simulink model "targetModel"  (R2016b)
settings: Solver=ode4  StartTime=0.0  StopTime=Inf  FixedStep=0.025  RelTol=1e-3  EnableMultiTasking=on
StartFcn:
  | fprintf('\nModel started\n')
  | % Change to root path of simulink model
  | %cd('C:\Users\Doctor V\Desktop\Water Channel Control2');
StopFcn:
  | fprintf('\nModel stopped, running callback.\n')
  | 
  | % change to the home directory
  | fprintf('\nChanging working directory to home directory.\n')
  | %cd('C:\Users\Doctor V\Desktop\Water Channel Control2');
  | 
  | % Add subdirectories to search path
  | fprintf('\nAdding subdirectories to search path.\n')
  | %addpath(genpath(pwd));
  | 
  | % Run stop script to save data and stuff.
  | fprintf('\nRunning stop script ".\\functions\\runAfterSim".\n')
  | %runAfterSim
model workspace (MAT data in the model file):
  Ts = 0.025
undefined symbols (not defined in the file or in its folder): acA2000, Ace, Basler, Freerun_FIX_YAW, PoCL
libraries: slrtlib x4, xpcbitflowlib x3, xpcvideoutillib x2, xpcnilib x1, xpcrtudplib x1
(part 1 of 3)
settings Model: xpc_rtwmakecfg_data=_jpeg__bitflow_  SimulationMode=external  Creator=gweast  LastModifiedBy=Doctor V
settings SolverCC: EnableConcurrentExecution=on
settings DataIOCC: MaxDataPoints=9999999999999999999999999999  SaveFormat=Array  SignalLoggingSaveFormat=ModelDataLogs  SaveState=on  SignalLogging=off  DSMLogging=off  VisualizeSimOutput=off
settings OptimizationCC: BlockReduction=off  OptimizeBlockIOStorage=off  BufferReuse=off  GlobalBufferReuse=off  ExpressionFolding=off  ExpressionDepthLimit=2147483647  LocalBlockOutputs=off  LifeSpan=inf  SimCompilerOptimization=on
settings DebuggingCC: UnderspecifiedInitializationDetection=Classic  MergeDetectMultiDrivingBlocksExec=none  SolverPrmCheckMsg=warning  FcnCallInpInsideContextMsg=warning  AllowSymbolicDim=off  StateNameClashWarn=warning  SFUnexpectedBacktrackingDiag=warning  SFNoUnconditionalDefaultTransitionDiag=warning  SFExecutionAtInitializationDiag=none
settings HardwareCC: ProdBitPerPointer=32  ProdBitPerSizeT=32  ProdBitPerPtrDiffT=32  ProdLargestAtomicFloat=None  ProdWordSize=32  ProdLongLongMode=on  ProdHWDeviceType=Generic->32-bit x86 compatible  TargetBitPerLong=64  TargetBitPerPointer=64  TargetIntDivRoundTo=Zero  TargetEndianess=LittleEndian  TargetWordSize=64  TargetHWDeviceType=Intel->x86-64
settings ModelReferenceCC: PropagateSignalLabelsOutOfModel=off
settings RTWCC: SystemTargetFile=slrt.tlc  TLCOptions=-axPCModelStackSizeKB=512  TemplateMakefile=slrt_default_tmf  Description=Simulink Real-Time  GenerateReport=on  RTWCompilerOptimization=on
settings ConfigComp: CovMetricSettings=dw  CovHtmlReporting=on  CovSaveCumulativeToWorkspaceVar=on  CovSaveSingleToWorkspaceVar=on  CovExternalEMLEnable=off

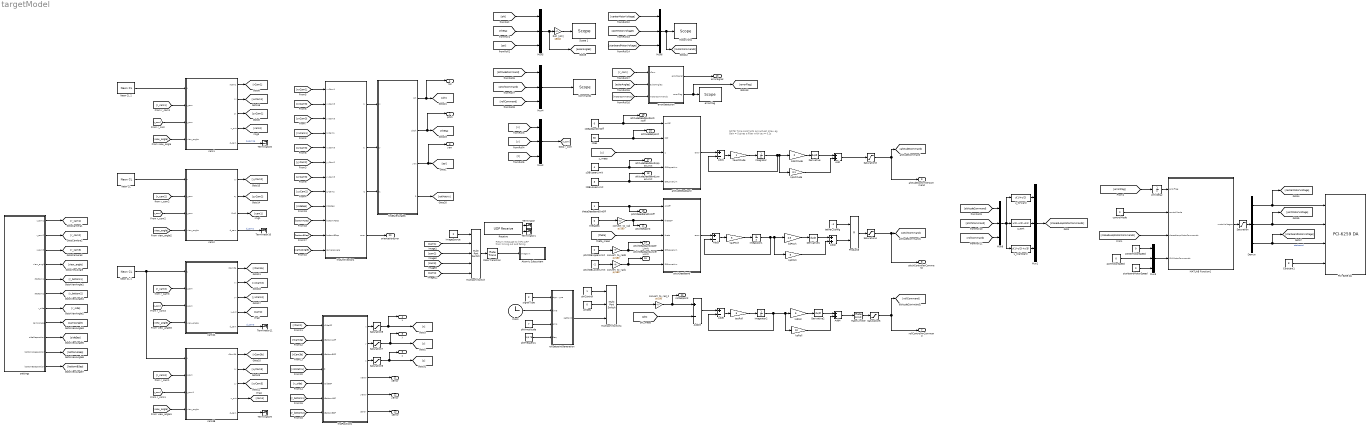
== system targetModel ==
  note: NOTE: Time constants are actuall 1/tau.
      | eg Gain = 5 gives a filter with tau = 0.2s
  note: Return message to keep ARP
      | from timing out and failing
  Add : Sum
  Add{1,3,5,19} (4 alike) : Sum  Inputs=+-
  Add2 : Sum
  Add4 : Sum
  Atomic Subsystem : Subsystem  TreatAsAtomicUnit=on  SystemSampleTime=Ts*3
  Clock : Clock
  Commands : slrtlib/Displays and Logging/Scope   Tag=Power Factor  Priority=1  scopeno=4  scopetype=Target  autostart=on  viewmode=Graphical rolling  formatstr='%15.6f'  grid=on  ylimits=[-1.65,1.65]  nosamples=400  noprepostsamples=0  interleave=1  triggermode=FreeRun  triggersignal=1  trigsignalfromport=off  triggerlevel=0.0  triggerslope=Either  triggerscope=1  triggersample=0  filename=data.dat  mode=Lazy  writesize=512  autorestart=off  dynamicfilemode=off  maxwritefilesize=512*1024^2
  Constant1 : Constant  Value=8
  Demux : Demux  Outputs=3
  Derivative : Derivative
  Derivative1 : Derivative
  Derivative2 : Derivative
  Integrator : Integrator
  Integrator1 : Integrator
  Integrator2 : Integrator
  MATLAB Function1 : MATLAB Function  TreatAsAtomicUnit=on
  "MotorVolts " : slrtlib/Displays and Logging/Scope   Tag=Motor Volts  Priority=2  scopeno=1  scopetype=Target  autostart=on  viewmode=Graphical rolling  formatstr='%15.6f'  grid=on  ylimits=[0,3.3]  nosamples=400  noprepostsamples=0  interleave=1  triggermode=FreeRun  triggersignal=1  trigsignalfromport=off  triggerlevel=0.0  triggerslope=Either  triggerscope=1  triggersample=0  filename=data.dat  mode=Lazy  writesize=512  autorestart=off  dynamicfilemode=off  maxwritefilesize=512*1024^2
  Multiport Switch : MultiPortSwitch  DataPortOrder=Zero-based contiguous  Inputs=4
  Multiport Switch4 : MultiPortSwitch  Inputs=2
  Mux{1..6,8} (7 alike) : Mux  Inputs=3
  "Neon CL " : xpcbitflowlib/Neon CL   camerapath=Basler-Ace-acA2000-340km-PoCL-3Tap-Freerun_FIX - ROLL.r64  r64=CAMERA  sampletime=-1  slot=[7,12]  make=Basler  model=acA2000-340km  mode=3 tap, 8-bits, 2040x1088 PoCL Free running  owner=BitFlow  revision=1  modelcomp=0  revcomp=0  aqtimeout=61440  format=1  flashmux=Mux_2TOEP  flashdcc=DCC  pixbitdepth=8  xsize=2040  ysize=1088  xstart=0  ystart=0  dx=2040  dy=1088  expmod="[0  0]"  config="[4294967295         128;4294967295           0;4294967295         512;4294967295           0;4294967295           0;4294967295           0;4294967295      262144;4294967295           0;4294967295           0;4294967295           0;4294967295     4195324;4294967295           0;4294967295           0;4294967295  4294967295;4294967295           0;4294967295           0;4294967295           0;4294967295    16777215;4294967295        1088;4294967295           0;4294967295           0;4294967295    16777215;4294967295           0;4294967295           0;4294967295           0;4294967295           0;4294967295           0;4294967295           0]"  ctab="[6      0     16      1  36880      2     16     96     18     97     16  32768      0]"  qtabmodel="[1   2040  65536]"  trigmode=0  baud=1  bytewidth=4  parity=1  stopbits=1  command="\"\""  response=0  comments=|
      | Three tap camera, 
      | Acquistion acquires 24 bits per clock, 
      | DMA works as 8-bit data
      | Set XSIZE = 3 * ACPL
  Neon CL 1 : xpcbitflowlib/Neon CL   camerapath=Basler-Ace-acA2000-340km-PoCL-3Tap-Freerun_FIX_YAW.r64  r64=CAMERA  sampletime=-1  slot=[4,12]  make=Basler  model=acA2000-340km  mode=3 tap, 8-bits, 2040x1088 PoCL Free running  owner=BitFlow  revision=1  modelcomp=0  revcomp=0  aqtimeout=61440  format=1  flashmux=Mux_2TOEP  flashdcc=DCC  pixbitdepth=8  xsize=2040  ysize=1088  xstart=0  ystart=0  dx=2040  dy=1088  expmod="[0  0]"  config="[4294967295         128;4294967295           0;4294967295         512;4294967295           0;4294967295           0;4294967295           0;4294967295      262144;4294967295           0;4294967295           0;4294967295           0;4294967295     4195324;4294967295           0;4294967295           0;4294967295  4294967295;4294967295           0;4294967295           0;4294967295           0;4294967295     4958209;4294967295        1088;4294967295           0;4294967295           0;4294967295  2164260863;4294967295           0;4294967295           0;4294967295           0;4294967295           0;4294967295     4958208;4294967295           0]"  ctab="[6      0     16      1  36880      2     16     96     18     97     16  32768      0]"  qtabmodel="[1   2040  65536]"  trigmode=0  baud=1  bytewidth=4  parity=1  stopbits=1  command="\"\""  response=0  comments=|
      | Three tap camera, 
      | Acquistion acquires 24 bits per clock, 
      | DMA works as 8-bit data
      | Set XSIZE = 3 * ACPL
  Neon CL 2 : xpcbitflowlib/Neon CL   camerapath=Basler-Ace-acA2000-340km-PoCL-3Tap-Freerun_FIX - PITCH.r64  r64=CAMERA  sampletime=-1  slot=[13,12]  make=Basler  model=acA2000-340km  mode=3 tap, 8-bits, 2040x1088 PoCL Free running  owner=BitFlow  revision=1  modelcomp=0  revcomp=0  aqtimeout=61440  format=1  flashmux=Mux_2TOEP  flashdcc=DCC  pixbitdepth=8  xsize=2040  ysize=1088  xstart=0  ystart=0  dx=2040  dy=1088  expmod="[0  0]"  config="[4294967295         128;4294967295           0;4294967295         512;4294967295           0;4294967295           0;4294967295           0;4294967295      262144;4294967295           0;4294967295           0;4294967295           0;4294967295     4195324;4294967295           0;4294967295           0;4294967295  4294967295;4294967295           0;4294967295           0;4294967295           0;4294967295     7528449;4294967295        1088;4294967295           0;4294967295           0;4294967295           0;4294967295           0;4294967295           0;4294967295           0;4294967295           0;4294967295     7528448;4294967295           0]"  ctab="[6      0     16      1  36880      2     16     96     18     97     16  32768      0]"  qtabmodel="[1   2040  65536]"  trigmode=0  baud=1  bytewidth=4  parity=1  stopbits=1  command="\"\""  response=0  comments=|
      | Three tap camera, 
      | Acquistion acquires 24 bits per clock, 
      | DMA works as 8-bit data
      | Set XSIZE = 3 * ACPL
  PCI-6259 DA : xpcnilib/D//A/M Series/PCI-6259 DA  channel=[1 2 3 4]  range=[5 10 5 10]  reset=[1 1 1 1]  initValue=[0 0 0 0]  sampletime=-1  slot=-1
  Product3 : Product
  Rate Limiter : RateLimiter  RisingSlewLimit=20  FallingSlewLimit=-20  SampleTimeMode=inherited
  Rate Transition : RateTransition
  Receive : xpcrtudplib/UDP Receive  ipAddressVal=Use host-target connection  localPort=25005  rcvWidth=1  rcvFmAny=off  fmAddress=10.10.10.10  sampleTime=Ts
  Roll_[phi] : Gain  Gain=180/pi
  Saturation : Saturate  UpperLimit=3.3  LowerLimit=0
  Saturation3 : Saturate  UpperLimit=1.65  LowerLimit=-1.65
  Saturation4 : Saturate  UpperLimit=1.65  LowerLimit=-1.65
  Saturation5 : Saturate  UpperLimit=1.65  LowerLimit=-1.65
  Saturation6 : Saturate  UpperLimit=90  LowerLimit=10
  Saturation7 : Saturate  UpperLimit=50  LowerLimit=-50
  Saturation8 : Saturate  UpperLimit=100  LowerLimit=-10
  Scope 1 : slrtlib/Displays and Logging/Scope   scopeno=5  scopetype=Target  autostart=on  viewmode=Graphical redraw  formatstr='%15.6f'  grid=on  ylimits=[0,0]  nosamples=250  noprepostsamples=0  interleave=1  triggermode=FreeRun  triggersignal=1  trigsignalfromport=off  triggerlevel=0.0  triggerslope=Either  triggerscope=1  triggersample=0  filename=data.dat  mode=Lazy  writesize=512  autorestart=off  dynamicfilemode=off  maxwritefilesize=512*1024^2
  Terminator{,1,8..11} (6 alike) : Terminator
  Unit Delay : UnitDelay  SampleTime=-1
  altitudeDeadband : MATLAB Function  TreatAsAtomicUnit=on
  cam1 : Subsystem
  cam2 : Subsystem
  cam3A : Subsystem
  cam3B : Subsystem
  centerMotorSpeed : Constant  Value=0
  controlMode : Constant  Value=0
  convert_to_rad : Gain  Gain=pi/180
  convert_to_rad1 : Gain  Gain=pi/180
  convert_to_rad3 : Gain  Gain=pi/180
  convert_to_rad_2 : Gain  Gain=pi/180
  errorDetection : MATLAB Function  TreatAsAtomicUnit=on
  errorFlag : slrtlib/Displays and Logging/Scope   Tag=Motor Volts  Priority=2  scopeno=2  scopetype=Target  autostart=on  viewmode=Graphical rolling  formatstr='%15.6f'  grid=on  ylimits=[0,2]  nosamples=400  noprepostsamples=0  interleave=1  triggermode=FreeRun  triggersignal=1  trigsignalfromport=off  triggerlevel=0.0  triggerslope=Either  triggerscope=1  triggersample=0  filename=data.dat  mode=Lazy  writesize=512  autorestart=off  dynamicfilemode=off  maxwritefilesize=512*1024^2
  findEulerAngles : MATLAB Function  TreatAsAtomicUnit=on
  findPositions : MATLAB Function  TreatAsAtomicUnit=on
  findUnitVectors : MATLAB Function  TreatAsAtomicUnit=on
  imageSource : Constant  Value=2
  kdAltitude : Gain  Gain=0
  kdPitch : Gain  Gain=2.5
  kdRoll : Gain  Gain=5
  kpAltitude : Gain  Gain=0.1
  kpPitch : Gain  Gain=5
  kpRoll : Gain  Gain=10
  phiAmplitude : Constant  Value=7
  phiControl : Constant
  phiDes : Constant  Value=0
  phiFrequency : Constant  Value=1/5.75
  pitchDBLowerLimit : Constant  Value=-2
  pitchDBUpperLimit : Constant  Value=2
  pitchDeadband : MATLAB Function  TreatAsAtomicUnit=on
  portMotorSpeed : Constant  Value=0
  rollSetpointGeneration : MATLAB Function  TreatAsAtomicUnit=on
  settings : Subsystem
  signalType : Constant  Value=2
  starboardMotorSpeed : Constant  Value=0
  tauAltitude : Gain
  tauPitch : Gain  Gain=5
  tauRoll : Gain  Gain=5
  tether_config : Constant  Value=-1
  thetaDeadbandOnOff : Constant
  thetaDes : Constant  Value=0
  u_forward : Fcn  Expr=u(1)+u(2)
  u_port : Fcn  Expr=u(1)-u(2)-u(3)
  u_starboard : Fcn  Expr=u(1)-u(2)+u(3)
  zDBLowerLimit : Constant  Value=3
  zDBUpperLimit : Constant  Value=4
  zDeadbandOnOff : Constant  Value=0
  zDes : Constant  Value=60
  roll : Outport
  pitch : Outport  Port=2
  yaw : Outport  Port=3
  x : Outport  Port=4
  y : Outport  Port=5
  z : Outport  Port=6
  rollControllerCommand : Outport  Port=7
  pitchControllerCommand : Outport  Port=8
  altitudeControllerCommand : Outport  Port=9
  altitudeSetpoint : Outport  Port=10
  pitchSetpoint : Outport  Port=11
  rollSetpoint : Outport  Port=12
  errorSignal : Outport  Port=13
  pitchDeadbandUpperLimit : Outport  Port=14
  pitchDeadbandLowerLimit : Outport  Port=15
  pitchDeadbandOnOff : Outport  Port=16
  altitudeDeadbandUpperLimit : Outport  Port=17
  altitudeDeadbandLowerLimit : Outport  Port=18
  altitudeDeadbandonOnOff : Outport  Port=19
  orientationError : Outport  Port=20
  xError : Outport  Port=21
  yError : Outport  Port=22
  zError : Outport  Port=23
  wires:
  Constant1/1 -> PCI-6259 DA/4
  controlMode/1 -> MATLAB Function1/2(controlMode)
  [phi] -> Add19/2
  [theta] -> pitchDeadband/3(theta)
  cam1/1(rCam1) -> [rCam1]
  cam3A/1(rCam3a) -> [rCam3a]
  Add19/1 -> Add5/1
  Demux/3 -> [starboardMotorVoltage], PCI-6259 DA/3  "starboard"
  Neon CL 1/1 -> cam3B/1(u), cam3A/1("u ")
  cam1/2(xx) -> [xxCam1]
  cam1/3(zx) -> [zxCam1]
  cam3A/2(xx) -> [xxCam3]
  cam3A/3(yx) -> [yxCam3]
  findEulerAngles/2(pitch) -> pitch/1, [theta]
  findEulerAngles/1(roll) -> roll/1, [phi]
  findPositions/2(y) -> Saturation7/1
  findEulerAngles/3(yaw) -> yaw/1, [psi]
  convert_to_rad_2/1 -> Add19/1, rollSetpoint/1
  findPositions/3(z) -> Saturation6/1
  findPositions/1(x) -> Saturation8/1
  Mux8/1 -> u_starboard/1, u_forward/1, u_port/1
  tether_config/1 -> Product3/1
  Product3/1 -> Saturation4/1
  cam3B/2(xy) -> [xyCam3]
  cam3B/3(yy) -> [yyCam3]
  cam2/1(yy) -> [yyCam2]
  cam2/2(zy) -> [zyCam2]
  Neon CL 2/1 -> cam1/1(u)
  cam3B/4("u_out ") -> [cam4]
  cam2/3(Out1) -> [cam1]
  "Neon CL "/1 -> cam2/1("u ")
  cam3A/4(u_out) -> [cam2]
  Mux5/1 -> [eulerAngles], Roll_[phi]/1
  settings/1(r_cam1) -> [r_cam1]
  settings/2("r_cam2 ") -> [r_cam2]
  settings/3(r_cam3) -> [r_cam3]
  [r_cam1] -> cam1/2(r_cam)
  [r_cam3] -> cam3B/2(r_cam)
  [r_cam2] -> cam2/2(r_cam)
  [r_cam3] -> cam3A/2(r_cam)
  [r_com] -> cam3B/3(r_com1)
  [r_com] -> cam2/3("r_com ")
  [r_com] -> cam3A/3("r_com ")
  [r_com] -> cam1/3(r_com)
  cam1/5(d_cam) -> Terminator8/1  "d_cam1a"
  cam2/4(d_cam) -> Terminator10/1  "d_cam2"
  cam3A/5(d_cam) -> Terminator11/1  "d_cam3"
  cam3B/5(d_cam) -> Terminator9/1
  settings/4(view_angle) -> [view_angle]
  [view_angle] -> cam1/4(view_angle)
  [view_angle] -> cam3B/4(view_angle)
  [view_angle] -> cam2/4(view_angle)
  [view_angle] -> cam3A/4(view_angle)
  cam1/4(u_out) -> [cam3]
  phiAmplitude/1 -> rollSetpointGeneration/3(amp)
  phiFrequency/1 -> rollSetpointGeneration/4(freq)
  Multiport Switch4/1 -> convert_to_rad_2/1
  rollSetpointGeneration/1(setPoint) -> Multiport Switch4/3
  phiDes/1 -> Multiport Switch4/2
  phiControl/1 -> Multiport Switch4/1
  thetaDes/1 -> convert_to_rad/1
  Clock/1 -> rollSetpointGeneration/2(time)
  portMotorSpeed/1 -> Mux3/2
  Mux3/1 -> MATLAB Function1/4(GUIMotorCommands)
  signalType/1 -> rollSetpointGeneration/1(signalType)
  Rate Limiter/1 -> Saturation5/1
  Saturation3/1 -> altitudeControllerCommand/1, [altitudeCommand]
  Saturation4/1 -> pitchControllerCommand/1, [pitchCommand]
  Saturation5/1 -> [rollCommand], rollControllerCommand/1
  zDes/1 -> altitudeDeadband/2(zSP), altitudeSetpoint/1
  u_forward/1 -> Mux1/1
  u_port/1 -> Mux1/2
  u_starboard/1 -> Mux1/3
  Mux1/1 -> [closedLoopMotorCommands]
  [closedLoopMotorCommands] -> MATLAB Function1/3(closedLoopMotorCommands)
  centerMotorSpeed/1 -> Mux3/1
  starboardMotorSpeed/1 -> Mux3/3
  MATLAB Function1/1(motorVoltages) -> Saturation/1
  [psi] -> Mux5/3
  [theta] -> Mux5/2
  [phi] -> Mux5/1
  [z] -> Mux2/3
  [y] -> Mux2/2
  [x] -> Mux2/1
  Mux2/1 -> [r_com]
  Saturation6/1 -> z/1, [z]
  Saturation7/1 -> [y], y/1
  Saturation8/1 -> x/1, [x]
  [rollCommand] -> Mux4/3
  [pitchCommand] -> Mux4/2
  [altitudeCommand] -> Mux4/1
  Mux4/1 -> Commands/1
  [rollCommand] -> Mux8/3
  [pitchCommand] -> Mux8/2
  [altitudeCommand] -> Mux8/1
  tauAltitude/1 -> Integrator/1
  kdAltitude/1 -> Derivative/1
  Integrator/1 -> Add1/2, kpAltitude/1, kdAltitude/1
  Derivative/1 -> Add/1
  kpAltitude/1 -> Add/2
  Add1/1 -> tauAltitude/1
  Add/1 -> Saturation3/1
  tauPitch/1 -> Integrator1/1
  kdPitch/1 -> Derivative1/1
  Integrator1/1 -> Add3/2, kpPitch/1, kdPitch/1
  Add2/1 -> Product3/2
  Derivative1/1 -> Add2/1
  kpPitch/1 -> Add2/2
  Add3/1 -> tauPitch/1
  tauRoll/1 -> Integrator2/1
  kdRoll/1 -> Derivative2/1
  Integrator2/1 -> Add5/2, kpRoll/1, kdRoll/1
  Add4/1 -> Rate Limiter/1
  Derivative2/1 -> Add4/1
  kpRoll/1 -> Add4/2
  Add5/1 -> tauRoll/1
  Saturation/1 -> Demux/1
  Demux/2 -> [portMotorVoltage], PCI-6259 DA/2
  Demux/1 -> [centerMotorVoltage], PCI-6259 DA/1
  [starboardMotorVoltage] -> Mux6/3
  [portMotorVoltage] -> Mux6/2
  [centerMotorVoltage] -> Mux6/1
  Mux6/1 -> [motorCommands], "MotorVolts "/1
  settings/5(rBottom1) -> [r_bottom1]
  settings/7(r_side) -> [r_side]
  [eulerAngles] -> errorDetection/2(eulerAngles)
  errorDetection/2(errorFlag) -> [errorFlag], errorFlag/1
  [motorCommands] -> errorDetection/3(motorCommands)
  [r_com] -> errorDetection/1(rCom)
  errorDetection/1(errorSignal) -> errorSignal/1
  pitchDeadband/1(error) -> Add3/1
  [errorFlag] -> Unit Delay/1
  convert_to_rad/1 -> pitchSetpoint/1, pitchDeadband/2(thetaSP)
  pitchDBUpperLimit/1 -> convert_to_rad3/1
  convert_to_rad3/1 -> pitchDeadband/4(DBUpperLim), pitchDeadbandUpperLimit/1
  Unit Delay/1 -> MATLAB Function1/1(errorFlag)
  pitchDBLowerLimit/1 -> convert_to_rad1/1
  convert_to_rad1/1 -> pitchDeadband/5(DBLowerLim), pitchDeadbandLowerLimit/1
  thetaDeadbandOnOff/1 -> pitchDeadbandOnOff/1, pitchDeadband/1(onOff)
  [z] -> altitudeDeadband/3(z)
  zDeadbandOnOff/1 -> altitudeDeadbandonOnOff/1, altitudeDeadband/1(onOff)
  zDBUpperLimit/1 -> altitudeDeadbandUpperLimit/1, altitudeDeadband/4(DBUpperLim)
  zDBLowerLimit/1 -> altitudeDeadbandLowerLimit/1, altitudeDeadband/5(DBLowerLim)
  altitudeDeadband/1(error) -> Add1/1
  [zyCam2] -> findUnitVectors/8(zyCam2)
  [xxCam1] -> findUnitVectors/1(xxCam1)
  [zxCam1] -> findUnitVectors/4(zxCam1)
  [xxCam3] -> findUnitVectors/2(xxCam3)
  [xyCam3] -> findUnitVectors/5(xyCam3)
  [yxCam3] -> findUnitVectors/3(yxCam3)
  [yyCam3] -> findUnitVectors/7(yyCam3)
  [yyCam2] -> findUnitVectors/6(yyCam2)
  [cam2Angle] -> findUnitVectors/12(cameraAngle)
  settings/8(cam2Angle) -> [cam2Angle]
  findUnitVectors/1(rx) -> findEulerAngles/1(rx)
  findUnitVectors/2(ry) -> findEulerAngles/2(ry)
  findUnitVectors/3(rz) -> findEulerAngles/3(rz)
  findUnitVectors/4(error) -> orientationError/1
  settings/6(rBottom2) -> [r_bottom2]
  cam3B/1(rCam3b) -> [rCam3b]
  [rCam1] -> findPositions/1(rSideGF)
  [rCam3a] -> findPositions/2(rBottomAGF)
  [rCam3b] -> findPositions/3(rBottomBGF)
  [r_side] -> findPositions/5(rSideBF)
  [r_bottom1] -> findPositions/6(rBottomABF)
  [r_bottom2] -> findPositions/7(rBottomBBF)
  findPositions/4(xError) -> xError/1
  findPositions/6(zError) -> zError/1
  findPositions/5(yError) -> yError/1
  [bottomBSep] -> findUnitVectors/11(bottomBSep)
  [bottomASep] -> findUnitVectors/10(bottomASep)
  [sideSep] -> findUnitVectors/9(sideSep)
  settings/9(sideSeparation) -> [sideSep]
  settings/10(bottomASeparation) -> [bottomASep]
  settings/11(bottomBSeparation) -> [bottomBSep]
  findEulerAngles/4(R) -> [rotMatrix]
  [rotMatrix] -> findPositions/4(R)
  Roll_[phi]/1 -> Scope 1/1
  Rate Transition/1 -> Atomic Subsystem/1(Image In)
  Receive/1 -> Terminator/1
  Receive/2 -> Terminator1/1
  imageSource/1 -> Multiport Switch/1
  [cam1] -> Multiport Switch/2
  [cam3] -> Multiport Switch/4
  [cam2] -> Multiport Switch/3
  Multiport Switch/1 -> Rate Transition/1
  [cam4] -> Multiport Switch/5

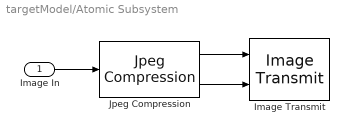
== system targetModel/Atomic Subsystem ==
  Image In : Inport
  Image Transmit : xpcvideoutillib/Image Transmit  ipAddress=255.255.255.255  ipPort=25000  localPort=-1  vblLen=on  maxpacket=40*1024  sampletime=-1
  Jpeg Compression : xpcvideoutillib/Jpeg Compression  quality=35  cspace=Grayscale  isig=One multidimensional signal  maxsize=2040*1088  length=on
  wires:
  Jpeg Compression/1 -> Image Transmit/1
  Jpeg Compression/2 -> Image Transmit/2
  Image In/1 -> Jpeg Compression/1

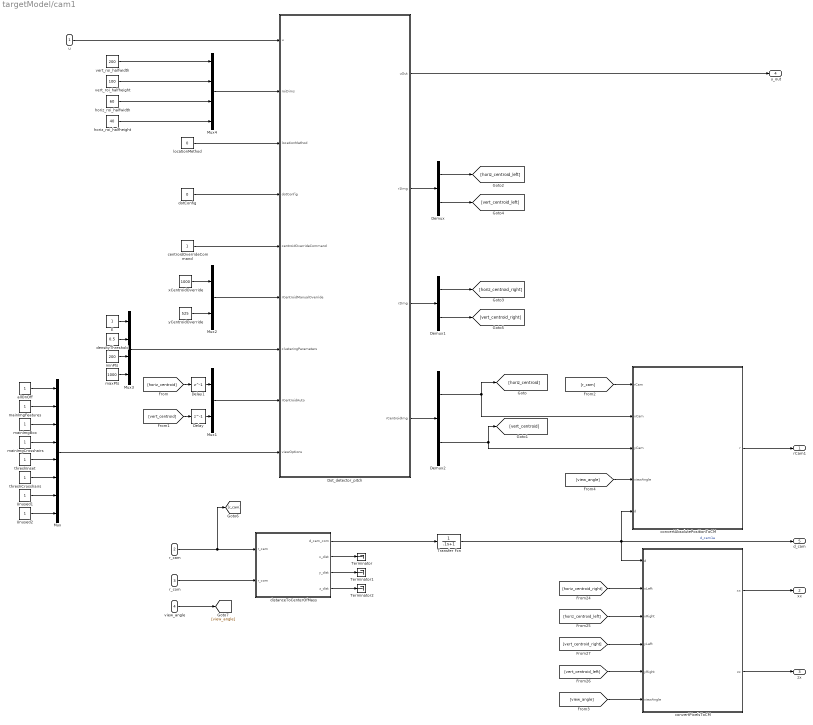
== system targetModel/cam1 ==
  u : Inport
  r_cam : Inport  Port=2
  r_com : Inport  Port=3
  view_angle : Inport  Port=4
  Delay : Delay  DelayLength=1  InitialCondition=800
  Delay1 : Delay  DelayLength=1  InitialCondition=1460
  Demux : Demux  Outputs=2
  Demux1 : Demux  Outputs=2
  Demux2 : Demux  Outputs=2
  Dot_detector_pitch : MATLAB Function  TreatAsAtomicUnit=on
  E : Constant
  Mux : Mux  Inputs=8
  Mux1 : Mux  Inputs=2
  Mux2 : Mux  Inputs=2
  Mux3 : Mux
  Mux4 : Mux
  Terminator : Terminator
  Terminator1 : Terminator
  Terminator2 : Terminator
  Transfer Fcn : TransferFcn  Denominator=[.1 1]
  Unused1 : Constant
  Unused2 : Constant
  allOnOff : Constant
  centroidOverrideCommand : Constant
  convertAbsolutePositionToCM : MATLAB Function  TreatAsAtomicUnit=on
  convertPixelsToCM : MATLAB Function  TreatAsAtomicUnit=on
  densityThreshold : Constant  Value=0.5
  distanceToCenterOfMass : MATLAB Function  TreatAsAtomicUnit=on
  dotConfig : Constant  Value=0
  horiz_roi_halfheight : Constant  Value=40
  horiz_roi_halfwidth : Constant  Value=60
  locationMethod : Constant  Value=0
  mainImgBox : Constant
  mainImgCrosshairs : Constant
  mainImgFeatures : Constant
  maxPts : Constant  Value=1000
  minPts : Constant  Value=200
  threshCrosshairs : Constant
  threshInset : Constant
  vert_roi_halfheight : Constant  Value=100
  vert_roi_halfwidth : Constant  Value=200
  xCentroidOverride : Constant  Value=1000
  yCentroidOverride : Constant  Value=525
  rCam1 : Outport
  xx : Outport  Port=2
  zx : Outport  Port=3
  u_out : Outport  Port=4
  d_cam : Outport  Port=5
  wires:
  [horiz_centroid] -> Delay1/1
  [vert_centroid] -> Delay/1
  allOnOff/1 -> Mux/1
  mainImgFeatures/1 -> Mux/2
  mainImgBox/1 -> Mux/3
  mainImgCrosshairs/1 -> Mux/4
  threshInset/1 -> Mux/5
  threshCrosshairs/1 -> Mux/6
  Unused1/1 -> Mux/7
  Unused2/1 -> Mux/8
  Dot_detector_pitch/1(uOut) -> u_out/1
  Mux1/1 -> Dot_detector_pitch/8(rCentroidAuto)
  Delay1/1 -> Mux1/1
  Delay/1 -> Mux1/2
  xCentroidOverride/1 -> Mux2/1
  yCentroidOverride/1 -> Mux2/2
  densityThreshold/1 -> Mux3/2
  minPts/1 -> Mux3/3
  maxPts/1 -> Mux3/4
  Mux3/1 -> Dot_detector_pitch/7(clusteringParameters)
  E/1 -> Mux3/1
  centroidOverrideCommand/1 -> Dot_detector_pitch/5(centroidOverrideCommand)
  Mux/1 -> Dot_detector_pitch/9(viewOptions)
  u/1 -> Dot_detector_pitch/1(u)
  Mux4/1 -> Dot_detector_pitch/2(roiDims)
  locationMethod/1 -> Dot_detector_pitch/3(locationMethod)
  dotConfig/1 -> Dot_detector_pitch/4(dotConfig)
  Demux/1 -> [horiz_centroid_left]
  Demux/2 -> [vert_centroid_left]
  Dot_detector_pitch/2(r1Img) -> Demux/1
  Dot_detector_pitch/3(r2Img) -> Demux1/1
  Demux1/1 -> [horiz_centroid_right]
  Demux1/2 -> [vert_centroid_right]
  Dot_detector_pitch/4(rCentroidImg) -> Demux2/1
  Demux2/1 -> convertAbsolutePositionToCM/2(xCam), [horiz_centroid]
  Demux2/2 -> convertAbsolutePositionToCM/3(yCam), [vert_centroid]
  Mux2/1 -> Dot_detector_pitch/6(rCentroidManualOverride)
  r_cam/1 -> [r_cam], distanceToCenterOfMass/1(r_cam)
  distanceToCenterOfMass/2(x_dist) -> Terminator/1
  distanceToCenterOfMass/3(y_dist) -> Terminator1/1
  distanceToCenterOfMass/4(z_dist) -> Terminator2/1
  [horiz_centroid_right] -> convertPixelsToCM/2(xLeft)
  [horiz_centroid_left] -> convertPixelsToCM/3(xRight)
  [vert_centroid_right] -> convertPixelsToCM/4(yLeft)
  [vert_centroid_left] -> convertPixelsToCM/5(yRight)
  convertPixelsToCM/1(xx) -> xx/1
  convertPixelsToCM/2(zx) -> zx/1
  r_com/1 -> distanceToCenterOfMass/2(r_com)
  distanceToCenterOfMass/1(d_cam_com) -> Transfer Fcn/1
  Transfer Fcn/1 -> convertAbsolutePositionToCM/5(d), convertPixelsToCM/1(d), d_cam/1  "d_cam1a"
  convertAbsolutePositionToCM/1(r) -> rCam1/1
  [r_cam] -> convertAbsolutePositionToCM/1(rCam)
  view_angle/1 -> [view_angle]
  [view_angle] -> convertPixelsToCM/6(viewAngle)
  [view_angle] -> convertAbsolutePositionToCM/4(viewAngle)
  vert_roi_halfwidth/1 -> Mux4/1
  horiz_roi_halfheight/1 -> Mux4/4
  vert_roi_halfheight/1 -> Mux4/2
  horiz_roi_halfwidth/1 -> Mux4/3

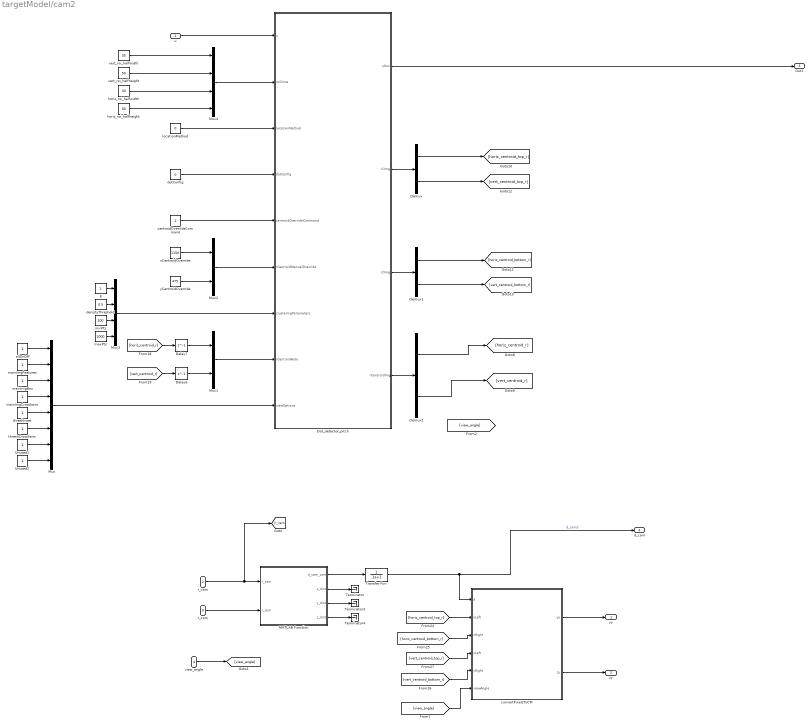
== system targetModel/cam2 ==
  "u " : Inport
  r_cam : Inport  Port=2
  "r_com " : Inport  Port=3
  view_angle : Inport  Port=4
  Delay6 : Delay  DelayLength=1  InitialCondition=800
  Delay7 : Delay  DelayLength=1  InitialCondition=1460
  Demux : Demux  Outputs=2
  Demux1 : Demux  Outputs=2
  Demux2 : Demux  Outputs=2
  Dot_detector_pitch : MATLAB Function  TreatAsAtomicUnit=on
  E : Constant
  MATLAB Function : MATLAB Function  TreatAsAtomicUnit=on
  Mux : Mux  Inputs=8
  Mux1 : Mux  Inputs=2
  Mux2 : Mux  Inputs=2
  Mux3 : Mux
  Mux4 : Mux
  Terminator : Terminator
  Terminator3 : Terminator
  Terminator4 : Terminator
  Transfer Fcn : TransferFcn  Denominator=[.1 1]
  Unused1 : Constant
  Unused2 : Constant
  allOnOff : Constant
  centroidOverrideCommand : Constant
  convertPixelsToCM : MATLAB Function  TreatAsAtomicUnit=on
  densityThreshold : Constant  Value=0.5
  dotConfig : Constant  Value=0
  horiz_roi_halfheight : Constant  Value=50
  horiz_roi_halfwidth : Constant  Value=30
  locationMethod : Constant  Value=0
  mainImgBox : Constant
  mainImgCrosshairs : Constant
  mainImgFeatures : Constant
  maxPts : Constant  Value=1000
  minPts : Constant  Value=200
  threshCrosshairs : Constant
  threshInset : Constant
  vert_roi_halfheight : Constant  Value=50
  vert_roi_halfwidth : Constant  Value=35
  xCentroidOverride : Constant  Value=1150
  yCentroidOverride : Constant  Value=475
  yy : Outport
  zy : Outport  Port=2
  Out1 : Outport  Port=3
  d_cam : Outport  Port=4
  wires:
  Demux/1 -> [horiz_centroid_top_r]
  Demux1/1 -> [horiz_centroid_bottom_r]
  Demux2/2 -> [vert_centroid_r]
  Demux1/2 -> [vert_centroid_bottom_r]
  Demux/2 -> [vert_centroid_top_r]
  [horiz_centroid_r] -> Delay7/1
  [vert_centroid_r] -> Delay6/1
  Mux1/1 -> Dot_detector_pitch/8(rCentroidAuto)
  xCentroidOverride/1 -> Mux2/1
  yCentroidOverride/1 -> Mux2/2
  densityThreshold/1 -> Mux3/2
  minPts/1 -> Mux3/3
  maxPts/1 -> Mux3/4
  Mux3/1 -> Dot_detector_pitch/7(clusteringParameters)
  E/1 -> Mux3/1
  centroidOverrideCommand/1 -> Dot_detector_pitch/5(centroidOverrideCommand)
  locationMethod/1 -> Dot_detector_pitch/3(locationMethod)
  dotConfig/1 -> Dot_detector_pitch/4(dotConfig)
  Dot_detector_pitch/2(r1Img) -> Demux/1
  Dot_detector_pitch/3(r2Img) -> Demux1/1
  Dot_detector_pitch/4(rCentroidImg) -> Demux2/1
  Mux2/1 -> Dot_detector_pitch/6(rCentroidManualOverride)
  Delay7/1 -> Mux1/1
  Delay6/1 -> Mux1/2
  allOnOff/1 -> Mux/1
  mainImgFeatures/1 -> Mux/2
  mainImgBox/1 -> Mux/3
  mainImgCrosshairs/1 -> Mux/4
  threshInset/1 -> Mux/5
  threshCrosshairs/1 -> Mux/6
  Unused1/1 -> Mux/7
  Unused2/1 -> Mux/8
  Mux/1 -> Dot_detector_pitch/9(viewOptions)
  Dot_detector_pitch/1(uOut) -> Out1/1
  "u "/1 -> Dot_detector_pitch/1(u)
  MATLAB Function/2(x_dist) -> Terminator/1
  MATLAB Function/3(y_dist) -> Terminator3/1
  MATLAB Function/4(z_dist) -> Terminator4/1
  r_cam/1 -> [r_cam], MATLAB Function/1(r_cam)
  "r_com "/1 -> MATLAB Function/2(r_com)
  MATLAB Function/1(d_cam_com) -> Transfer Fcn/1
  Transfer Fcn/1 -> convertPixelsToCM/1(d), d_cam/1  "d_cam2"
  [horiz_centroid_top_r] -> convertPixelsToCM/2(xLeft)
  [horiz_centroid_bottom_r] -> convertPixelsToCM/3(xRight)
  [vert_centroid_top_r] -> convertPixelsToCM/4(yLeft)
  [vert_centroid_bottom_r] -> convertPixelsToCM/5(yRight)
  convertPixelsToCM/1(yy) -> yy/1
  convertPixelsToCM/2(zy) -> zy/1
  Demux2/1 -> [horiz_centroid_r]
  view_angle/1 -> [view_angle]
  [view_angle] -> convertPixelsToCM/6(viewAngle)
  Mux4/1 -> Dot_detector_pitch/2(roiDims)
  vert_roi_halfwidth/1 -> Mux4/1
  horiz_roi_halfheight/1 -> Mux4/4
  vert_roi_halfheight/1 -> Mux4/2
  horiz_roi_halfwidth/1 -> Mux4/3

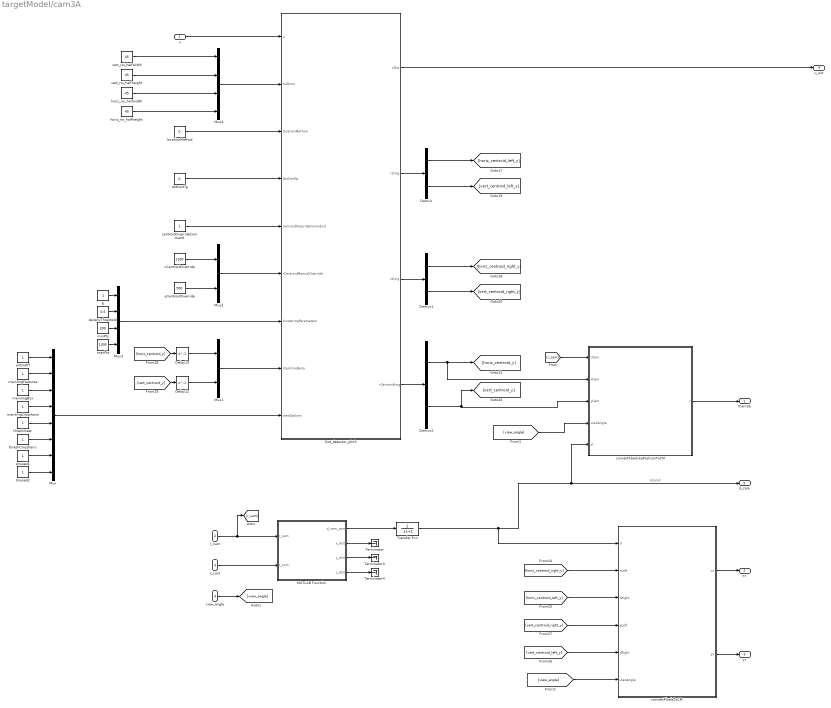
== system targetModel/cam3A ==
  "u " : Inport
  r_cam : Inport  Port=2
  "r_com " : Inport  Port=3
  view_angle : Inport  Port=4
  Delay12 : Delay  DelayLength=1  InitialCondition=800
  Delay13 : Delay  DelayLength=1  InitialCondition=1460
  Demux : Demux  Outputs=2
  Demux1 : Demux  Outputs=2
  Demux2 : Demux  Outputs=2
  Dot_detector_pitch : MATLAB Function  TreatAsAtomicUnit=on
  E : Constant
  MATLAB Function : MATLAB Function  TreatAsAtomicUnit=on
  Mux : Mux  Inputs=8
  Mux1 : Mux  Inputs=2
  Mux2 : Mux  Inputs=2
  Mux3 : Mux
  Mux4 : Mux
  Terminator : Terminator
  Terminator3 : Terminator
  Terminator4 : Terminator
  Transfer Fcn : TransferFcn  Denominator=[.1 1]
  Unused1 : Constant
  Unused2 : Constant
  allOnOff : Constant
  centroidOverrideCommand : Constant
  convertAbsolutePositionToCM : MATLAB Function  TreatAsAtomicUnit=on
  convertPixelsToCM : MATLAB Function  TreatAsAtomicUnit=on
  densityThreshold : Constant  Value=0.5
  dotConfig : Constant  Value=0
  horiz_roi_halfheight : Constant  Value=45
  horiz_roi_halfwidth : Constant  Value=45
  locationMethod : Constant  Value=0
  mainImgBox : Constant
  mainImgCrosshairs : Constant
  mainImgFeatures : Constant
  maxPts : Constant  Value=1000
  minPts : Constant  Value=200
  threshCrosshairs : Constant
  threshInset : Constant
  vert_roi_halfheight : Constant  Value=45
  vert_roi_halfwidth : Constant  Value=45
  xCentroidOverride : Constant  Value=1100
  yCentroidOverride : Constant  Value=500
  rCam3a : Outport
  xx : Outport  Port=2
  yx : Outport  Port=3
  u_out : Outport  Port=4
  d_cam : Outport  Port=5
  wires:
  [vert_centroid_y] -> Delay12/1
  [horiz_centroid_y] -> Delay13/1
  Mux1/1 -> Dot_detector_pitch/8(rCentroidAuto)
  xCentroidOverride/1 -> Mux2/1
  yCentroidOverride/1 -> Mux2/2
  densityThreshold/1 -> Mux3/2
  minPts/1 -> Mux3/3
  maxPts/1 -> Mux3/4
  Mux3/1 -> Dot_detector_pitch/7(clusteringParameters)
  E/1 -> Mux3/1
  centroidOverrideCommand/1 -> Dot_detector_pitch/5(centroidOverrideCommand)
  locationMethod/1 -> Dot_detector_pitch/3(locationMethod)
  dotConfig/1 -> Dot_detector_pitch/4(dotConfig)
  Dot_detector_pitch/2(r1Img) -> Demux/1
  Dot_detector_pitch/3(r2Img) -> Demux1/1
  Dot_detector_pitch/4(rCentroidImg) -> Demux2/1
  Mux2/1 -> Dot_detector_pitch/6(rCentroidManualOverride)
  allOnOff/1 -> Mux/1
  mainImgFeatures/1 -> Mux/2
  mainImgBox/1 -> Mux/3
  mainImgCrosshairs/1 -> Mux/4
  threshInset/1 -> Mux/5
  threshCrosshairs/1 -> Mux/6
  Unused1/1 -> Mux/7
  Unused2/1 -> Mux/8
  Mux/1 -> Dot_detector_pitch/9(viewOptions)
  "u "/1 -> Dot_detector_pitch/1(u)
  Delay13/1 -> Mux1/1
  Delay12/1 -> Mux1/2
  Demux1/1 -> [horiz_centroid_right_y]
  Demux1/2 -> [vert_centroid_right_y]
  Demux/2 -> [vert_centroid_left_y]
  Demux/1 -> [horiz_centroid_left_y]
  Dot_detector_pitch/1(uOut) -> u_out/1
  Demux2/1 -> convertAbsolutePositionToCM/2(xCam), [horiz_centroid_y]
  MATLAB Function/2(x_dist) -> Terminator/1
  MATLAB Function/3(y_dist) -> Terminator3/1
  MATLAB Function/4(z_dist) -> Terminator4/1
  r_cam/1 -> [r_cam], MATLAB Function/1(r_cam)
  "r_com "/1 -> MATLAB Function/2(r_com)
  MATLAB Function/1(d_cam_com) -> Transfer Fcn/1
  Transfer Fcn/1 -> convertPixelsToCM/1(d), convertAbsolutePositionToCM/5(d), d_cam/1  "dcam3"
  [horiz_centroid_right_y] -> convertPixelsToCM/2(xLeft)
  [horiz_centroid_left_y] -> convertPixelsToCM/3(xRight)
  [vert_centroid_right_y] -> convertPixelsToCM/4(yLeft)
  [vert_centroid_left_y] -> convertPixelsToCM/5(yRight)
  convertPixelsToCM/1(xx) -> xx/1
  convertPixelsToCM/2(yx) -> yx/1
  Demux2/2 -> [vert_centroid_y], convertAbsolutePositionToCM/3(yCam)
  [r_cam] -> convertAbsolutePositionToCM/1(rCam)
  convertAbsolutePositionToCM/1(r) -> rCam3a/1
  view_angle/1 -> [view_angle]
  [view_angle] -> convertAbsolutePositionToCM/4(viewAngle)
  [view_angle] -> convertPixelsToCM/6(viewAngle)
  Mux4/1 -> Dot_detector_pitch/2(roiDims)
  vert_roi_halfwidth/1 -> Mux4/1
  horiz_roi_halfheight/1 -> Mux4/4
  vert_roi_halfheight/1 -> Mux4/2
  horiz_roi_halfwidth/1 -> Mux4/3

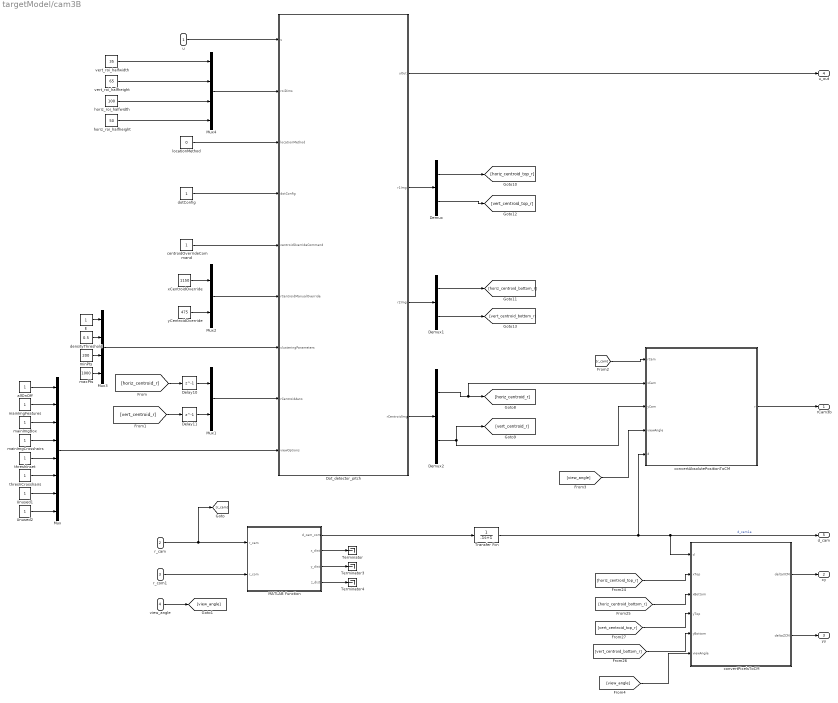
== system targetModel/cam3B ==
  u : Inport
  r_cam : Inport  Port=2
  r_com1 : Inport  Port=3
  view_angle : Inport  Port=4
  Delay10 : Delay  DelayLength=1  InitialCondition=1655
  Delay11 : Delay  DelayLength=1  InitialCondition=800
  Demux : Demux  Outputs=2
  Demux1 : Demux  Outputs=2
  Demux2 : Demux  Outputs=2
  Dot_detector_pitch : MATLAB Function  TreatAsAtomicUnit=on
  E : Constant
  MATLAB Function : MATLAB Function  TreatAsAtomicUnit=on
  Mux : Mux  Inputs=8
  Mux1 : Mux  Inputs=2
  Mux2 : Mux  Inputs=2
  Mux3 : Mux
  Mux4 : Mux
  Terminator : Terminator
  Terminator3 : Terminator
  Terminator4 : Terminator
  Transfer Fcn : TransferFcn  Denominator=[.1 1]
  Unused1 : Constant
  Unused2 : Constant
  allOnOff : Constant
  centroidOverrideCommand : Constant
  convertAbsolutePositionToCM : MATLAB Function  TreatAsAtomicUnit=on
  convertPixelsToCM : MATLAB Function  TreatAsAtomicUnit=on
  densityThreshold : Constant  Value=0.5
  dotConfig : Constant
  horiz_roi_halfheight : Constant  Value=50
  horiz_roi_halfwidth : Constant  Value=100
  locationMethod : Constant  Value=0
  mainImgBox : Constant
  mainImgCrosshairs : Constant
  mainImgFeatures : Constant
  maxPts : Constant  Value=1000
  minPts : Constant  Value=200
  threshCrosshairs : Constant
  threshInset : Constant
  vert_roi_halfheight : Constant  Value=65
  vert_roi_halfwidth : Constant  Value=35
  xCentroidOverride : Constant  Value=1150
  yCentroidOverride : Constant  Value=475
  rCam3b : Outport
  xy : Outport  Port=2
  yy : Outport  Port=3
  "u_out " : Outport  Port=4
  d_cam : Outport  Port=5
  wires:
  [vert_centroid_r] -> Delay11/1
  [horiz_centroid_r] -> Delay10/1
  allOnOff/1 -> Mux/1
  mainImgFeatures/1 -> Mux/2
  mainImgBox/1 -> Mux/3
  mainImgCrosshairs/1 -> Mux/4
  threshInset/1 -> Mux/5
  threshCrosshairs/1 -> Mux/6
  Unused1/1 -> Mux/7
  Unused2/1 -> Mux/8
  Mux1/1 -> Dot_detector_pitch/8(rCentroidAuto)
  xCentroidOverride/1 -> Mux2/1
  yCentroidOverride/1 -> Mux2/2
  densityThreshold/1 -> Mux3/2
  minPts/1 -> Mux3/3
  maxPts/1 -> Mux3/4
  Mux3/1 -> Dot_detector_pitch/7(clusteringParameters)
  E/1 -> Mux3/1
  centroidOverrideCommand/1 -> Dot_detector_pitch/5(centroidOverrideCommand)
  Mux/1 -> Dot_detector_pitch/9(viewOptions)
  u/1 -> Dot_detector_pitch/1(u)
  locationMethod/1 -> Dot_detector_pitch/3(locationMethod)
  dotConfig/1 -> Dot_detector_pitch/4(dotConfig)
  Dot_detector_pitch/2(r1Img) -> Demux/1
  Dot_detector_pitch/3(r2Img) -> Demux1/1
  Dot_detector_pitch/4(rCentroidImg) -> Demux2/1
  Mux2/1 -> Dot_detector_pitch/6(rCentroidManualOverride)
  Delay10/1 -> Mux1/1
  Delay11/1 -> Mux1/2
  Demux/1 -> [horiz_centroid_top_r]
  Demux/2 -> [vert_centroid_top_r]
  Demux1/1 -> [horiz_centroid_bottom_r]
  Demux1/2 -> [vert_centroid_bottom_r]
  Dot_detector_pitch/1(uOut) -> "u_out "/1
  Demux2/2 -> [vert_centroid_r], convertAbsolutePositionToCM/3(yCam)
  Demux2/1 -> convertAbsolutePositionToCM/2(xCam), [horiz_centroid_r]
  MATLAB Function/2(x_dist) -> Terminator/1
  MATLAB Function/3(y_dist) -> Terminator3/1
  MATLAB Function/4(z_dist) -> Terminator4/1
  r_cam/1 -> [r_cam], MATLAB Function/1(r_cam)
  r_com1/1 -> MATLAB Function/2(r_com)
  [horiz_centroid_top_r] -> convertPixelsToCM/2(xTop)
  [horiz_centroid_bottom_r] -> convertPixelsToCM/3(xBottom)
  [vert_centroid_top_r] -> convertPixelsToCM/4(yTop)
  [vert_centroid_bottom_r] -> convertPixelsToCM/5(yBottom)
  Transfer Fcn/1 -> convertAbsolutePositionToCM/5(d), convertPixelsToCM/1(d), d_cam/1  "d_cam1a"
  MATLAB Function/1(d_cam_com) -> Transfer Fcn/1
  convertPixelsToCM/2(deltaZCM) -> yy/1
  convertPixelsToCM/1(deltaXCM) -> xy/1
  [r_cam] -> convertAbsolutePositionToCM/1(rCam)
  convertAbsolutePositionToCM/1(r) -> rCam3b/1
  view_angle/1 -> [view_angle]
  [view_angle] -> convertAbsolutePositionToCM/4(viewAngle)
  [view_angle] -> convertPixelsToCM/6(viewAngle)
  Mux4/1 -> Dot_detector_pitch/2(roiDims)
  vert_roi_halfwidth/1 -> Mux4/1
  horiz_roi_halfheight/1 -> Mux4/4
  vert_roi_halfheight/1 -> Mux4/2
  horiz_roi_halfwidth/1 -> Mux4/3

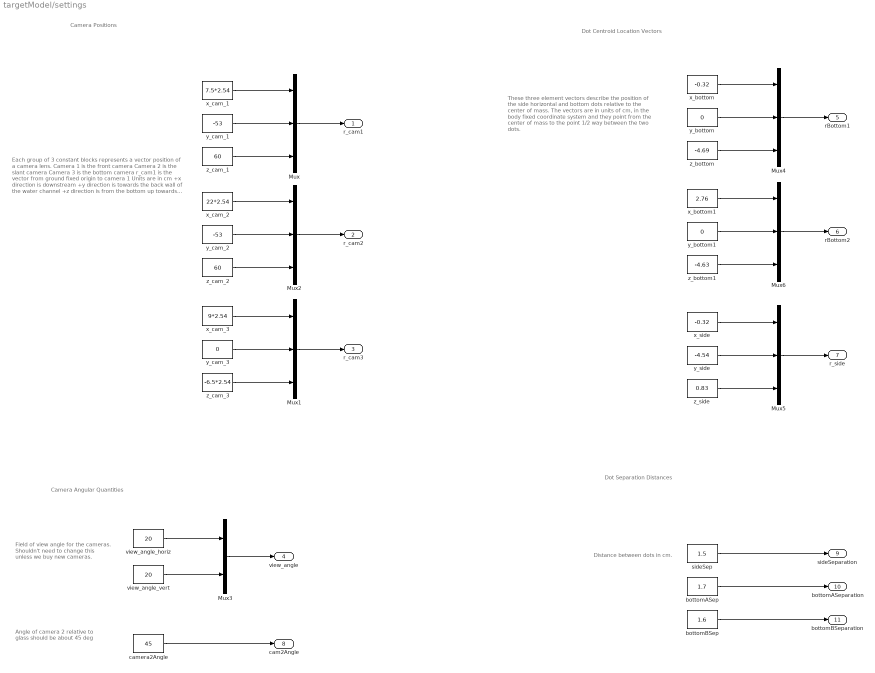
== system targetModel/settings ==
  note: Field of view angle
      | for the cameras.
      | Shouldn't need to change
      | this unless we buy new cameras.
  note: Camera Angular Quantities
  note: Dot Separation Distances
  note: Dot Centroid Location Vectors
  note: Camera Positions
  note: Distance between dots
      | in cm.
  note: Angle of camera 2
      | relative to glass
      | should be about
      | 45 deg
  note: These three element vectors describe the
      | position of the side horizontal and bottom dots
      | relative to the center of mass.  The vectors are in
      | units of cm, in the body fixed coordinate system and
      | they point from the center of mass to the point 1/2
      | way between the two dots.
  note: Each group of 3 constant
      | blocks represents a vector position of a camera lens.
      |
      | Camera 1 is the front camera
      | Camera 2 is the slant camera
      | Camera 3 is the bottom camera
      |
      | r_cam1 is the vector from ground fixed origin to camera 1
      |
      | Units are in cm
      | +x direction is downstream
      | +y direction is towards the back wall of the water channel
      | +z direction is from the bottom up towards the water surface
  Mux{,1..2,4..6} (6 alike) : Mux  Inputs=3
  Mux3 : Mux  Inputs=2
  bottomASep : Constant  Value=1.7
  bottomBSep : Constant  Value=1.6
  camera2Angle : Constant  Value=45
  sideSep : Constant  Value=1.5
  view_angle_horiz : Constant  Value=20
  view_angle_vert : Constant  Value=20
  x_bottom : Constant  Value=-0.32
  x_bottom1 : Constant  Value=2.76
  x_cam_1 : Constant  Value=7.5*2.54
  x_cam_2 : Constant  Value=22*2.54
  x_cam_3 : Constant  Value=9*2.54
  x_side : Constant  Value=-0.32
  y_bottom : Constant  Value=0
  y_bottom1 : Constant  Value=0
  y_cam_1 : Constant  Value=-53
  y_cam_2 : Constant  Value=-53
  y_cam_3 : Constant  Value=0
  y_side : Constant  Value=-4.54
  z_bottom : Constant  Value=-4.69
  z_bottom1 : Constant  Value=-4.63
  z_cam_1 : Constant  Value=60
  z_cam_2 : Constant  Value=60
  z_cam_3 : Constant  Value=-6.5*2.54
  z_side : Constant  Value=0.83
  r_cam1 : Outport
  "r_cam2 " : Outport  Port=2
  r_cam3 : Outport  Port=3
  view_angle : Outport  Port=4
  rBottom1 : Outport  Port=5
  rBottom2 : Outport  Port=6
  r_side : Outport  Port=7
  cam2Angle : Outport  Port=8
  sideSeparation : Outport  Port=9
  bottomASeparation : Outport  Port=10
  bottomBSeparation : Outport  Port=11
  wires:
  x_cam_1/1 -> Mux/1
  y_cam_1/1 -> Mux/2
  z_cam_1/1 -> Mux/3
  Mux/1 -> r_cam1/1
  x_cam_2/1 -> Mux2/1
  y_cam_2/1 -> Mux2/2
  z_cam_2/1 -> Mux2/3
  x_cam_3/1 -> Mux1/1
  y_cam_3/1 -> Mux1/2
  z_cam_3/1 -> Mux1/3
  Mux2/1 -> "r_cam2 "/1
  Mux1/1 -> r_cam3/1
  view_angle_horiz/1 -> Mux3/1
  view_angle_vert/1 -> Mux3/2
  Mux3/1 -> view_angle/1
  y_bottom/1 -> Mux4/2
  z_bottom/1 -> Mux4/3
  Mux4/1 -> rBottom1/1
  x_bottom/1 -> Mux4/1
  y_side/1 -> Mux5/2
  z_side/1 -> Mux5/3
  Mux5/1 -> r_side/1
  x_side/1 -> Mux5/1
  camera2Angle/1 -> cam2Angle/1
  y_bottom1/1 -> Mux6/2
  z_bottom1/1 -> Mux6/3
  Mux6/1 -> rBottom2/1
  x_bottom1/1 -> Mux6/1
  bottomASep/1 -> bottomASeparation/1
  bottomBSep/1 -> bottomBSeparation/1
  sideSep/1 -> sideSeparation/1
